simulink model "sim_tcyb_2023_obs"  (R2020a)
settings: Solver=ode4  StartTime=0.0  StopTime=30.0  FixedStep=0.01  RelTol=1e-3
values from neighbouring files (symbols this model uses):
  b1 = 6.0    (= 6)    [init_tcyb_2023_obs.m]
  c1 = 6.0    (= 6)    [init_tcyb_2023_obs.m]
  delta1 = 0.1    [init_tcyb_2023_obs.m]
  delta2 = 0.1    [init_tcyb_2023_obs.m]
  k0 = 2    [init_tcyb_2023_obs.m]
  kai_1_t = 0.02    [init_tcyb_2023_obs.m]
  kai_3_t = 0.1    [init_tcyb_2023_obs.m]
  lambda_max_P = max(eig(Pij))    [init_tcyb_2023_obs.m]
  lambda_min_Q = min(eig(Qij))    [init_tcyb_2023_obs.m]
  Mii = diag([1;0;0;0;1])    [init_tcyb_2023_obs.m]
  pos0 = zeros(3, 1)    [init_tcyb_2023_obs.m]
  PZ0 = P0(3)    [init_tcyb_2023_obs.m]
  PZ1 = 10    [init_tcyb_2023_obs.m]
  R0 = 4    [init_tcyb_2023_obs.m]
  R1 = 8    [init_tcyb_2023_obs.m]
  Rx2 = 10    [init_tcyb_2023_obs.m]
  Ry2 = 6    [init_tcyb_2023_obs.m]
  Rz2 = 4    [init_tcyb_2023_obs.m]
  T0 = 0    [init_tcyb_2023_obs.m]
  T1 = tseq1    (= 10)    [init_tcyb_2023_obs.m]
  T12 = tseq1 + tseq12    (= 20)    [init_tcyb_2023_obs.m]
  T2 = tseq1 + tseq12 + tseq2    (= 30)    [init_tcyb_2023_obs.m]
  theta0 = ( 2 / 5 ) * pi    (= 1.25663706144)    [init_tcyb_2023_obs.m]
  ts1 = 10    [init_tcyb_2023_obs.m]
  ts2 = 20    [init_tcyb_2023_obs.m]
  vel0 = zeros(3, 1)    [init_tcyb_2023_obs.m]
  Wij = [0,0,1,0,0;              0,0,1,1,0;              1,0,0,0,1;              0,1,1,0,0;              0,0,1,0,0]    [init_tcyb_2023_obs.m]
  X1 = 8    [init_tcyb_2023_obs.m]
  X2 = 2    [init_tcyb_2023_obs.m]
  X3 = 3    [init_tcyb_2023_obs.m]
  Y1 = 10    [init_tcyb_2023_obs.m]
  Y2 = 2    [init_tcyb_2023_obs.m]
  Y3 = 4    [init_tcyb_2023_obs.m]
  Z1 = 4    [init_tcyb_2023_obs.m]
  Z2 = -6    [init_tcyb_2023_obs.m]
  Z3 = 2    [init_tcyb_2023_obs.m]
(part 2 of 2)

== matlab function sim_tcyb_2023_obs/process velocity ==
  data: T0 input; T1 input; T2 input; PZ0 input; PZ1 input; R0 input; R1 input; Rx2 input; Ry2 input; Rz2 input; t input; V_init_out output
function V_init_out = fcn(T0, T1, T2, PZ0, PZ1, R0, R1, Rx2, Ry2, Rz2, t)
V_init_out = zeros(3, 1);
if t < T1 + 1e-05
    V_init_out(1, 1) = ( cos( ( 2 * pi * ( t - T0 ) ) / ( T0 - T1 ) ) * ( R0 - R1 ) ) / ( T0 - T1 ) ...
                                    - ( 2 * pi * sin( ( 2 * pi * ( t - T0 ) ) / ( T0 - T1 ) ) * ( R0 + ( ( R0 - R1 ) * ( t - T0 ) ) / ( T0 - T1 ) ) ) / ( T0 - T1 );
    V_init_out(2, 1) = ( sin( ( 2 * pi * ( t - T0 ) ) / ( T0 - T1 ) ) * ( R0 - R1 ) ) / ( T0 - T1 ) ...
                                    + ( 2 * pi * cos( ( 2 * pi * ( t - T0 ) ) / ( T0 - T1 ) ) * ( R0 + ( ( R0 - R1 ) * ( t - T0 ) ) / ( T0 - T1 ) ) ) / ( T0 - T1 );
    V_init_out(3, 1) = ( PZ0 - PZ1 ) / ( T0 - T1 );
else
    V_init_out(1, 1) = ( 2 * Rx2 * pi * sin( ( 2 * pi * ( t - T1 ) ) / ( T1 - T2 ) ) ) / ( T1 - T2 );
    V_init_out(2, 1) = ( 4 * Ry2 * pi * cos( ( 4 * pi * ( t - T1 ) ) / ( T1 - T2 ) ) ) / ( T1 - T2 );
    V_init_out(3, 1) = - ( 4 * Rz2 * pi * cos( ( 4 * pi * ( t - T1 ) ) / ( T1 - T2 ) ) ) / ( T1 - T2 );
end
